simulink model "mrefrobotarm_modified_previous_y_previous_u_previous_ref_pert"  (R2018b)
settings: Solver=FixedStepAuto  StartTime=0.0  StopTime=10  RelTol=1e-3  AbsTol=1e-6
undefined symbols (not defined in the file or in its folder): cc, options
libraries: neural x714, simulink x1
(part 6 of 26)

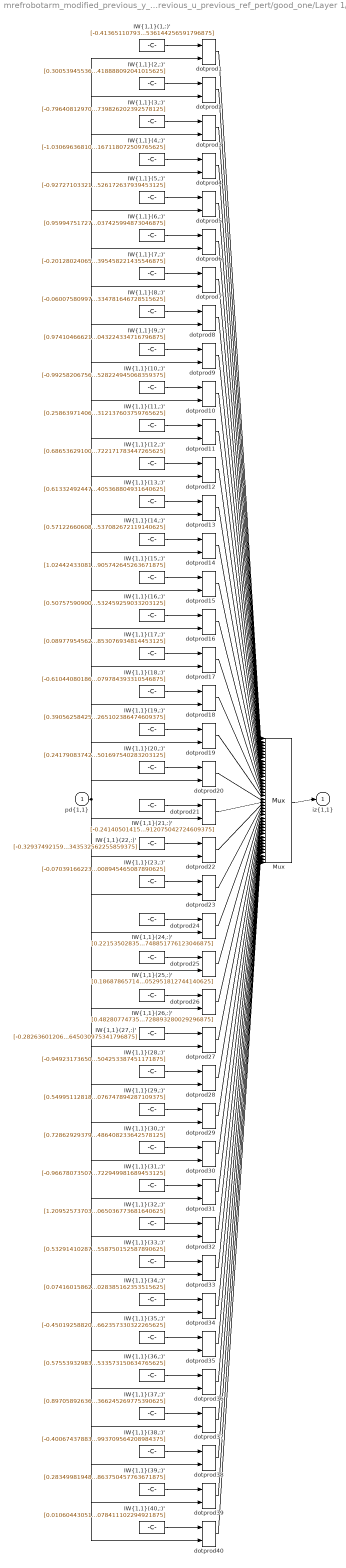
== system mrefrobotarm_modified_previous_y_previous_u_previous_ref_pert/good_one/Layer 1/IW{1,1} ==
  "pd{1,1}" : Inport  PortDimensions=10
      mask Display: e = 0.06;c1 = [120 230 180]/255;c2 = ([120 230 180]+0)/(256+128);c3 = ([120 230 180]+128)/(256+128);patch([0 1 1 0],[0 0 1 1],c1);patch([0 1 1 1-e 1-e 0+e],[0 0 1 1-e 0+e 0+e],c2);patch([0 0 1 1-e 0+e 0+e],[0 1 1 1-e 1-e 0+e],c3);plot([0 1 1 0 0],[0 0 1 1 0]);
  "IW{1,1}(1,:)'" : Constant  Value=[-0.413651107935018635952673093925113789737224578857421875;0.3836269510828476114738805335946381092071533203125;0.50232710069936759023079275721102021634578704833984375;-1.000665970829996087587687725317664444446563720703125;-0.1542635339068328670375507272183313034474849700927734375;-0.8218009806009398676707178310607559978961944580078125;-0.417486068359214090861541990307159721851348876953125;0.867526729012368047477821164648048579692840576171875;-0.98301388214653051544900108638103120028972625732421875;-0.0193724473873694395809064161539936321787536144256591796875]
      mask Display: e = 0.06;c1 = [120 150 230]/255;c2 = ([120 150 230]+0)/383;c3 = ([120 150 230]+128)/383;patch([0 1 1 0],[0 0 1 1],c1);patch([0 1 1 1-e 1-e 0+e],[0 0 1 1-e 0+e 0+e],c2);patch([0 0 1 1-e 0+e 0+e],[0 1 1 1-e 1-e 0+e],c3);plot([0 1 1 0 0],[0 0 1 1 0]);disp('Weights');
  "IW{1,1}(10,:)'" : Constant  Value=[-0.9925820675659589031880614129477180540561676025390625;0.2409702921885312765226672127027995884418487548828125;0.052011920879238393577992383143282495439052581787109375;-0.416376750462584432899149078366463072597980499267578125;-0.96039113919741703195853688157512806355953216552734375;0.62063415478920413992369731204234994947910308837890625;-0.8630530306659343064978884285665117204189300537109375;0.60936291205421666550279269358725287020206451416015625;-0.09827055594646873226682970425827079452574253082275390625;0.488985628143102812881437557734898291528224945068359375]
      mask Display: e = 0.06;c1 = [120 150 230]/255;c2 = ([120 150 230]+0)/383;c3 = ([120 150 230]+128)/383;patch([0 1 1 0],[0 0 1 1],c1);patch([0 1 1 1-e 1-e 0+e],[0 0 1 1-e 0+e 0+e],c2);patch([0 0 1 1-e 0+e 0+e],[0 1 1 1-e 1-e 0+e],c3);plot([0 1 1 0 0],[0 0 1 1 0]);disp('Weights');
  "IW{1,1}(11,:)'" : Constant  Value=[0.2586397140629539403988701451453380286693572998046875;-0.82856549831495229785360834284801967442035675048828125;0.6264712959270088976637680389103479683399200439453125;0.75547506719408696884698883877717889845371246337890625;0.59640906838833218639450706177740357816219329833984375;-0.785029365476563878445404043304733932018280029296875;-0.347310950192660339297390237334184348583221435546875;-0.462157651619720721836159782469621859490871429443359375;-1.1325499249033577076062329069827683269977569580078125;0.3696119827837540672277327757910825312137603759765625]
      mask Display: e = 0.06;c1 = [120 150 230]/255;c2 = ([120 150 230]+0)/383;c3 = ([120 150 230]+128)/383;patch([0 1 1 0],[0 0 1 1],c1);patch([0 1 1 1-e 1-e 0+e],[0 0 1 1-e 0+e 0+e],c2);patch([0 0 1 1-e 0+e 0+e],[0 1 1 1-e 1-e 0+e],c3);plot([0 1 1 0 0],[0 0 1 1 0]);disp('Weights');
  "IW{1,1}(12,:)'" : Constant  Value=[0.68653629100552582276151269979891367256641387939453125;-0.0248886322461292323893200517659352044574916362762451171875;0.447180501328404200744870422568055801093578338623046875;-0.44198123420568524721829817281104624271392822265625;-1.2490651394449863165192482483689673244953155517578125;0.4830653108523133010265837583574466407299041748046875;-0.392759951245398808428177517271251417696475982666015625;0.1335766512357776936159581282481667585670948028564453125;-0.583482604222464118493007845245301723480224609375;0.500678183603759041631064974353648722171783447265625]
      mask Display: e = 0.06;c1 = [120 150 230]/255;c2 = ([120 150 230]+0)/383;c3 = ([120 150 230]+128)/383;patch([0 1 1 0],[0 0 1 1],c1);patch([0 1 1 1-e 1-e 0+e],[0 0 1 1-e 0+e 0+e],c2);patch([0 0 1 1-e 0+e 0+e],[0 1 1 1-e 1-e 0+e],c3);plot([0 1 1 0 0],[0 0 1 1 0]);disp('Weights');
  "IW{1,1}(13,:)'" : Constant  Value=[0.6133249244779575004571370300254784524440765380859375;0.2368863057068739952359948119919863529503345489501953125;-0.826730624883238451872102814377285540103912353515625;-0.81502965756012690778931073509738780558109283447265625;0.049822669627226069677394804102732450701296329498291015625;0.49182006191557137153580470112501643598079681396484375;0.067178707635307921552936250009224750101566314697265625;0.145702225927659856363760582098620943725109100341796875;0.230253060188553015930068568195565603673458099365234375;1.0194493979983862974592057071276940405368804931640625]
      mask Display: e = 0.06;c1 = [120 150 230]/255;c2 = ([120 150 230]+0)/383;c3 = ([120 150 230]+128)/383;patch([0 1 1 0],[0 0 1 1],c1);patch([0 1 1 1-e 1-e 0+e],[0 0 1 1-e 0+e 0+e],c2);patch([0 0 1 1-e 0+e 0+e],[0 1 1 1-e 1-e 0+e],c3);plot([0 1 1 0 0],[0 0 1 1 0]);disp('Weights');
  "IW{1,1}(14,:)'" : Constant  Value=[0.57122660608382125335680257194326259195804595947265625;-0.70113249391813214916879815064021386206150054931640625;-0.0086478499608871224613171335704464581795036792755126953125;0.5990449634267556167088741858606226742267608642578125;-0.0532433606170133189028348397187073715031147003173828125;0.95479246182017474264824841156951151788234710693359375;-0.67799642096428913706773755620815791189670562744140625;0.157662545375461260466209978403639979660511016845703125;0.47531924881363696311353805867838673293590545654296875;1.1223503909760312868826304111280478537082672119140625]
      mask Display: e = 0.06;c1 = [120 150 230]/255;c2 = ([120 150 230]+0)/383;c3 = ([120 150 230]+128)/383;patch([0 1 1 0],[0 0 1 1],c1);patch([0 1 1 1-e 1-e 0+e],[0 0 1 1-e 0+e 0+e],c2);patch([0 0 1 1-e 0+e 0+e],[0 1 1 1-e 1-e 0+e],c3);plot([0 1 1 0 0],[0 0 1 1 0]);disp('Weights');
  "IW{1,1}(15,:)'" : Constant  Value=[1.024424330811316341538486085482873022556304931640625;-0.11900181038713032732889729459202499128878116607666015625;-0.89301318009671770692392556156846694648265838623046875;0.286811956595100336908643612332525663077831268310546875;0.9562237123416152950738933213870041072368621826171875;0.66112349620669796923522198994760401546955108642578125;0.65942560869206012785781467755441553890705108642578125;-0.3635154948717345124720168314524926245212554931640625;-0.12615629404641903743566899720462970435619354248046875;0.1510476304024055138608417792056570760905742645263671875]
      mask Display: e = 0.06;c1 = [120 150 230]/255;c2 = ([120 150 230]+0)/383;c3 = ([120 150 230]+128)/383;patch([0 1 1 0],[0 0 1 1],c1);patch([0 1 1 1-e 1-e 0+e],[0 0 1 1-e 0+e 0+e],c2);patch([0 0 1 1-e 0+e 0+e],[0 1 1 1-e 1-e 0+e],c3);plot([0 1 1 0 0],[0 0 1 1 0]);disp('Weights');
  "IW{1,1}(16,:)'" : Constant  Value=[0.50757590900584437232367918113595806062221527099609375;-0.68550796743866182492155303407344035804271697998046875;0.845989680309202629615583646227605640888214111328125;-0.301001414510317422124074937528348527848720550537109375;-0.5131342658860080785387935975450091063976287841796875;0.55499089075900476242253489544964395463466644287109375;0.87265805917673666680656197058851830661296844482421875;0.56120439816466494153957000889931805431842803955078125;0.3991413846511429053265374022885225713253021240234375;0.58399825658444382003864348007482476532459259033203125]
      mask Display: e = 0.06;c1 = [120 150 230]/255;c2 = ([120 150 230]+0)/383;c3 = ([120 150 230]+128)/383;patch([0 1 1 0],[0 0 1 1],c1);patch([0 1 1 1-e 1-e 0+e],[0 0 1 1-e 0+e 0+e],c2);patch([0 0 1 1-e 0+e 0+e],[0 1 1 1-e 1-e 0+e],c3);plot([0 1 1 0 0],[0 0 1 1 0]);disp('Weights');
  "IW{1,1}(17,:)'" : Constant  Value=[0.08977954562821359452140512757978285662829875946044921875;0.450162042402085627035290826825075782835483551025390625;-0.277132842312844906995650262615527026355266571044921875;-0.89533484630924953240338481919025070965290069580078125;0.48814571614230484186691683134995400905609130859375;-0.62095272399335910140649730237782932817935943603515625;-0.45038353462766200774325398015207611024379730224609375;-0.49284862337333013027063088884460739791393280029296875;0.760357222341462968273617661907337605953216552734375;0.70640094347899140547752949714777059853076934814453125]
      mask Display: e = 0.06;c1 = [120 150 230]/255;c2 = ([120 150 230]+0)/383;c3 = ([120 150 230]+128)/383;patch([0 1 1 0],[0 0 1 1],c1);patch([0 1 1 1-e 1-e 0+e],[0 0 1 1-e 0+e 0+e],c2);patch([0 0 1 1-e 0+e 0+e],[0 1 1 1-e 1-e 0+e],c3);plot([0 1 1 0 0],[0 0 1 1 0]);disp('Weights');
  "IW{1,1}(18,:)'" : Constant  Value=[-0.6104408018694840176721072566579096019268035888671875;-1.0336913526824804687720416040974669158458709716796875;0.270725265822102378887592522005434148013591766357421875;-0.380750786613607061781294760294258594512939453125;0.33268512528966043273470631902455352246761322021484375;-1.001093745459246786566609443980269134044647216796875;0.158315525907221921197987057894351892173290252685546875;-0.53153054346245409700344453085563145577907562255859375;-0.7668902743210084249625424490659497678279876708984375;-0.16671042993793416808756546743097715079784393310546875]
      mask Display: e = 0.06;c1 = [120 150 230]/255;c2 = ([120 150 230]+0)/383;c3 = ([120 150 230]+128)/383;patch([0 1 1 0],[0 0 1 1],c1);patch([0 1 1 1-e 1-e 0+e],[0 0 1 1-e 0+e 0+e],c2);patch([0 0 1 1-e 0+e 0+e],[0 1 1 1-e 1-e 0+e],c3);plot([0 1 1 0 0],[0 0 1 1 0]);disp('Weights');
  "IW{1,1}(19,:)'" : Constant  Value=[0.3905625842580298101580638103769160807132720947265625;0.0308098706564870587765181397799096885137259960174560546875;0.062138100461527102924552679041880764998495578765869140625;0.622615013248140058976787258870899677276611328125;0.99643920501872529360554153754492290318012237548828125;0.618145409712675064639597621862776577472686767578125;-1.1790025687618210792351192139904014766216278076171875;0.43713177654620272161167804370052181184291839599609375;-0.1320814385678981406346821358965826220810413360595703125;0.63245679741952220975775844635791145265102386474609375]
      mask Display: e = 0.06;c1 = [120 150 230]/255;c2 = ([120 150 230]+0)/383;c3 = ([120 150 230]+128)/383;patch([0 1 1 0],[0 0 1 1],c1);patch([0 1 1 1-e 1-e 0+e],[0 0 1 1-e 0+e 0+e],c2);patch([0 0 1 1-e 0+e 0+e],[0 1 1 1-e 1-e 0+e],c3);plot([0 1 1 0 0],[0 0 1 1 0]);disp('Weights');
  "IW{1,1}(2,:)'" : Constant  Value=[0.30053945536555570772208056951058097183704376220703125;0.481520714463711529962353097289451397955417633056640625;0.32855722206039239541297547475551255047321319580078125;-1.023620353434349983245965631795115768909454345703125;0.36139385403812862573857955794665031135082244873046875;-0.35510074464173346786566298760590143501758575439453125;0.53901574191551049342052692736615426838397979736328125;1.1478171331129953802729914968949742615222930908203125;0.01330999643922634555204265183192546828649938106536865234375;-0.8531970477840273847647267757565714418888092041015625]
      mask Display: e = 0.06;c1 = [120 150 230]/255;c2 = ([120 150 230]+0)/383;c3 = ([120 150 230]+128)/383;patch([0 1 1 0],[0 0 1 1],c1);patch([0 1 1 1-e 1-e 0+e],[0 0 1 1-e 0+e 0+e],c2);patch([0 0 1 1-e 0+e 0+e],[0 1 1 1-e 1-e 0+e],c3);plot([0 1 1 0 0],[0 0 1 1 0]);disp('Weights');
  "IW{1,1}(20,:)'" : Constant  Value=[0.2417908374206110544424319641620968468487262725830078125;-0.00914807597982341021147778548083806526847183704376220703125;0.084217128377931993465921323149814270436763763427734375;0.42983285451377406527484481557621620595455169677734375;1.3394232861488226671298207293148152530193328857421875;-0.381148886874808578983930829053861089050769805908203125;-0.1762973437296376510996509523465647362172603607177734375;0.09308197699677267511475520223029889166355133056640625;0.92227381408703601461951393503113649785518646240234375;1.077442550129131593195097593707032501697540283203125]
      mask Display: e = 0.06;c1 = [120 150 230]/255;c2 = ([120 150 230]+0)/383;c3 = ([120 150 230]+128)/383;patch([0 1 1 0],[0 0 1 1],c1);patch([0 1 1 1-e 1-e 0+e],[0 0 1 1-e 0+e 0+e],c2);patch([0 0 1 1-e 0+e 0+e],[0 1 1 1-e 1-e 0+e],c3);plot([0 1 1 0 0],[0 0 1 1 0]);disp('Weights');
  "IW{1,1}(21,:)'" : Constant  Value=[-0.2414050141565159679490903954501845873892307281494140625;0.82367477414810907898612413191585801541805267333984375;-0.0105825294795365530686748201105729094706475734710693359375;0.1956113083766050919631851456870208494365215301513671875;-1.7069096984195322175281717136385850608348846435546875;1.0057780668058187156788108040927909314632415771484375;1.4591709688934726418807485970319248735904693603515625;-0.2593923279024730188524472396238707005977630615234375;0.41043551676310585651918927396764047443866729736328125;0.83741947098360502987901554661220870912075042724609375]
      mask Display: e = 0.06;c1 = [120 150 230]/255;c2 = ([120 150 230]+0)/383;c3 = ([120 150 230]+128)/383;patch([0 1 1 0],[0 0 1 1],c1);patch([0 1 1 1-e 1-e 0+e],[0 0 1 1-e 0+e 0+e],c2);patch([0 0 1 1-e 0+e 0+e],[0 1 1 1-e 1-e 0+e],c3);plot([0 1 1 0 0],[0 0 1 1 0]);disp('Weights');
  "IW{1,1}(22,:)'" : Constant  Value=[-0.32937492159880077391420627463958226144313812255859375;0.646622243844576782834110417752526700496673583984375;-0.02931361877227912915433449825286515988409519195556640625;0.436759612951945042080836856257519684731960296630859375;0.866285245725330721455748061998747289180755615234375;0.1793659302452613457656838136244914494454860687255859375;0.09031635641268757896948926600089180283248424530029296875;-0.5973200815445045552820602097199298441410064697265625;0.10267351667025111094933009781016153283417224884033203125;1.2656338190569369483995387781760655343532562255859375]
      mask Display: e = 0.06;c1 = [120 150 230]/255;c2 = ([120 150 230]+0)/383;c3 = ([120 150 230]+128)/383;patch([0 1 1 0],[0 0 1 1],c1);patch([0 1 1 1-e 1-e 0+e],[0 0 1 1-e 0+e 0+e],c2);patch([0 0 1 1-e 0+e 0+e],[0 1 1 1-e 1-e 0+e],c3);plot([0 1 1 0 0],[0 0 1 1 0]);disp('Weights');
  "IW{1,1}(23,:)'" : Constant  Value=[-0.0703916622397355862261747461161576211452484130859375;0.67191045082923650522133129925350658595561981201171875;-0.0242859635021656396214329021177036338485777378082275390625;-0.386628048517191180710739217829541303217411041259765625;-2.5074712136418124686088049202226102352142333984375;0.55235033890016993485261309615452773869037628173828125;0.74299364405580725634337113660876639187335968017578125;0.64206786309071850471497100443230010569095611572265625;-0.58043464748950912568403737168409861624240875244140625;-0.422889498711053912760604589493595995008945465087890625]
      mask Display: e = 0.06;c1 = [120 150 230]/255;c2 = ([120 150 230]+0)/383;c3 = ([120 150 230]+128)/383;patch([0 1 1 0],[0 0 1 1],c1);patch([0 1 1 1-e 1-e 0+e],[0 0 1 1-e 0+e 0+e],c2);patch([0 0 1 1-e 0+e 0+e],[0 1 1 1-e 1-e 0+e],c3);plot([0 1 1 0 0],[0 0 1 1 0]);disp('Weights');
  "IW{1,1}(24,:)'" : Constant  Value=[0.221535028351505680621613691982929594814777374267578125;-0.8698822208881937800839523333706893026828765869140625;-0.2182601953161487917665084523832774721086025238037109375;0.4079298497457213290573463382315821945667266845703125;-0.36144550181965640067716094563365913927555084228515625;-0.28639131544193630052319576861918903887271881103515625;0.9540574961812564591667751301429234445095062255859375;-0.28396445607271247890679433112381957471370697021484375;0.364127425092508449910866374921170063316822052001953125;-0.004278262852394447250670150850737627479247748851776123046875]
      mask Display: e = 0.06;c1 = [120 150 230]/255;c2 = ([120 150 230]+0)/383;c3 = ([120 150 230]+128)/383;patch([0 1 1 0],[0 0 1 1],c1);patch([0 1 1 1-e 1-e 0+e],[0 0 1 1-e 0+e 0+e],c2);patch([0 0 1 1-e 0+e 0+e],[0 1 1 1-e 1-e 0+e],c3);plot([0 1 1 0 0],[0 0 1 1 0]);disp('Weights');
  "IW{1,1}(25,:)'" : Constant  Value=[0.186878657149024240968770982362912036478519439697265625;-0.7759331943091141159385415448923595249652862548828125;0.2148465953621268298423530040963669307529926300048828125;-0.92201175425662285078942659310996532440185546875;0.59498484563237952205128067362238653004169464111328125;-0.66139341790903605211582316769636236131191253662109375;0.67596601108655107736922218464314937591552734375;-0.458533778996277507911116799732553772628307342529296875;-0.322071301367099327439547096219030208885669708251953125;0.8937721561967253425251556109287776052951812744140625]
      mask Display: e = 0.06;c1 = [120 150 230]/255;c2 = ([120 150 230]+0)/383;c3 = ([120 150 230]+128)/383;patch([0 1 1 0],[0 0 1 1],c1);patch([0 1 1 1-e 1-e 0+e],[0 0 1 1-e 0+e 0+e],c2);patch([0 0 1 1-e 0+e 0+e],[0 1 1 1-e 1-e 0+e],c3);plot([0 1 1 0 0],[0 0 1 1 0]);disp('Weights');
  "IW{1,1}(26,:)'" : Constant  Value=[0.482807747351104932231891098126652650535106658935546875;-0.274643538698023714772489256574772298336029052734375;0.977117390542808994524648369406349956989288330078125;-0.72784044851192764014058411703445017337799072265625;-0.298911347579471187163591139324125833809375762939453125;-0.351550652031840493716430273707373999059200286865234375;-0.7121513278393643009422930845175869762897491455078125;0.94265145728446686490542560932226479053497314453125;-0.63767361421792767561811388077330775558948516845703125;-0.465068595673045592775451950728893280029296875]
      mask Display: e = 0.06;c1 = [120 150 230]/255;c2 = ([120 150 230]+0)/383;c3 = ([120 150 230]+128)/383;patch([0 1 1 0],[0 0 1 1],c1);patch([0 1 1 1-e 1-e 0+e],[0 0 1 1-e 0+e 0+e],c2);patch([0 0 1 1-e 0+e 0+e],[0 1 1 1-e 1-e 0+e],c3);plot([0 1 1 0 0],[0 0 1 1 0]);disp('Weights');
  "IW{1,1}(27,:)'" : Constant  Value=[-0.2826360120640381001777541314368136227130889892578125;1.0331384188045353855756047778413631021976470947265625;0.2538275640105565056359182563028298318386077880859375;-0.6876811465011194446361741938744671642780303955078125;0.4368710842237082392358615834382362663745880126953125;0.476320854183213071575409003344248048961162567138671875;0.443648508004234332080528702135779894888401031494140625;-0.62347776206357463646412497837445698678493499755859375;0.43560219075936379429236922078416682779788970947265625;0.6740756065088635562432273218291811645030975341796875]
      mask Display: e = 0.06;c1 = [120 150 230]/255;c2 = ([120 150 230]+0)/383;c3 = ([120 150 230]+128)/383;patch([0 1 1 0],[0 0 1 1],c1);patch([0 1 1 1-e 1-e 0+e],[0 0 1 1-e 0+e 0+e],c2);patch([0 0 1 1-e 0+e 0+e],[0 1 1 1-e 1-e 0+e],c3);plot([0 1 1 0 0],[0 0 1 1 0]);disp('Weights');
  "IW{1,1}(28,:)'" : Constant  Value=[-0.94923173650253056532477557993843220174312591552734375;-0.98442046864123933236356833731406368315219879150390625;0.41376330233902114397182003813213668763637542724609375;0.439113670992825666505865456201718188822269439697265625;0.21542815920926638995069879456423223018646240234375;-0.93574938767304816078507201382308267056941986083984375;0.787753205288106439496687016799114644527435302734375;-0.226104675231449281369577875011600553989410400390625;0.048265716907905320542937488426105119287967681884765625;0.54952586236559042287552756533841602504253387451171875]
      mask Display: e = 0.06;c1 = [120 150 230]/255;c2 = ([120 150 230]+0)/383;c3 = ([120 150 230]+128)/383;patch([0 1 1 0],[0 0 1 1],c1);patch([0 1 1 1-e 1-e 0+e],[0 0 1 1-e 0+e 0+e],c2);patch([0 0 1 1-e 0+e 0+e],[0 1 1 1-e 1-e 0+e],c3);plot([0 1 1 0 0],[0 0 1 1 0]);disp('Weights');
  "IW{1,1}(29,:)'" : Constant  Value=[0.54995112818424851663934305179282091557979583740234375;-0.96548476888214762592355100423446856439113616943359375;-0.6133643858887316557826352436677552759647369384765625;-0.369747278830332037902195452261366881430149078369140625;-0.4889943619153596099380365558317862451076507568359375;-0.4574687563627983788450137581094168126583099365234375;-0.9918414740130405693463444549706764519214630126953125;-0.439705044341271389374270484040607698261737823486328125;0.5677934762199841056684590512304566800594329833984375;-0.5441783375664319688524983575916849076747894287109375]
      mask Display: e = 0.06;c1 = [120 150 230]/255;c2 = ([120 150 230]+0)/383;c3 = ([120 150 230]+128)/383;patch([0 1 1 0],[0 0 1 1],c1);patch([0 1 1 1-e 1-e 0+e],[0 0 1 1-e 0+e 0+e],c2);patch([0 0 1 1-e 0+e 0+e],[0 1 1 1-e 1-e 0+e],c3);plot([0 1 1 0 0],[0 0 1 1 0]);disp('Weights');
  "IW{1,1}(3,:)'" : Constant  Value=[-0.79640812970941443627026501417276449501514434814453125;-0.96725622206039030270829925939324311912059783935546875;-0.81005379713580738521017110542743466794490814208984375;0.07789219319437627742086505122642847709357738494873046875;-0.86489171738730241667525433513219468295574188232421875;0.81312859030495265866278487010276876389980316162109375;-0.12379626000382269734867435317937633953988552093505859375;-0.6992501943224880278648925013840198516845703125;-0.0202103147915163768033597335715967346914112567901611328125;0.4651949651069664515290469353203661739826202392578125]
      mask Display: e = 0.06;c1 = [120 150 230]/255;c2 = ([120 150 230]+0)/383;c3 = ([120 150 230]+128)/383;patch([0 1 1 0],[0 0 1 1],c1);patch([0 1 1 1-e 1-e 0+e],[0 0 1 1-e 0+e 0+e],c2);patch([0 0 1 1-e 0+e 0+e],[0 1 1 1-e 1-e 0+e],c3);plot([0 1 1 0 0],[0 0 1 1 0]);disp('Weights');
  "IW{1,1}(30,:)'" : Constant  Value=[0.72862929379874075141998446270008571445941925048828125;0.57099515174563386654682517473702318966388702392578125;-0.09992527021377718698946779340985813178122043609619140625;0.411812398181885364056853404690627939999103546142578125;-1.1646039332940241184388696638052351772785186767578125;-0.81635251644773576540359272257774136960506439208984375;-0.1168473553190165492576824135539936833083629608154296875;-0.359766465525852507933990409583202563226222991943359375;0.6195063284556125982049934464157558977603912353515625;0.038312220849707818992602170737882261164486408233642578125]
      mask Display: e = 0.06;c1 = [120 150 230]/255;c2 = ([120 150 230]+0)/383;c3 = ([120 150 230]+128)/383;patch([0 1 1 0],[0 0 1 1],c1);patch([0 1 1 1-e 1-e 0+e],[0 0 1 1-e 0+e 0+e],c2);patch([0 0 1 1-e 0+e 0+e],[0 1 1 1-e 1-e 0+e],c3);plot([0 1 1 0 0],[0 0 1 1 0]);disp('Weights');
  "IW{1,1}(31,:)'" : Constant  Value=[-0.96678073507359851834763730948907323181629180908203125;0.09148655759019690136835123439595918171107769012451171875;0.709549141602580757393070598482154309749603271484375;-0.410248808800185826850537296195398084819316864013671875;-0.7370652145869300841951599068124778568744659423828125;-0.438942207461164246584672810058691538870334625244140625;-0.80989777442946098151566047818050719797611236572265625;0.94874940597907764239238304071477614343166351318359375;0.2334139145840961881983588455113931559026241302490234375;0.405630960838893106501501506500062532722949981689453125]
      mask Display: e = 0.06;c1 = [120 150 230]/255;c2 = ([120 150 230]+0)/383;c3 = ([120 150 230]+128)/383;patch([0 1 1 0],[0 0 1 1],c1);patch([0 1 1 1-e 1-e 0+e],[0 0 1 1-e 0+e 0+e],c2);patch([0 0 1 1-e 0+e 0+e],[0 1 1 1-e 1-e 0+e],c3);plot([0 1 1 0 0],[0 0 1 1 0]);disp('Weights');
  "IW{1,1}(32,:)'" : Constant  Value=[1.2095257370328458268460281033185310661792755126953125;0.35065561767196407050306561359320767223834991455078125;-0.95698055747720101038567008799873292446136474609375;-0.18743931116112688695096721858135424554347991943359375;-1.0822736049319747753116871535894460976123809814453125;1.075874990384995566472525752033106982707977294921875;-0.352754600872055512628122642126982100307941436767578125;0.314480530229425181421021306960028596222400665283203125;-1.20745251513363083262220243341289460659027099609375;0.134532970678878316395099545843550004065036773681640625]
      mask Display: e = 0.06;c1 = [120 150 230]/255;c2 = ([120 150 230]+0)/383;c3 = ([120 150 230]+128)/383;patch([0 1 1 0],[0 0 1 1],c1);patch([0 1 1 1-e 1-e 0+e],[0 0 1 1-e 0+e 0+e],c2);patch([0 0 1 1-e 0+e 0+e],[0 1 1 1-e 1-e 0+e],c3);plot([0 1 1 0 0],[0 0 1 1 0]);disp('Weights');
  "IW{1,1}(33,:)'" : Constant  Value=[0.532914102879858742056740084080956876277923583984375;1.105100254369091317130369134247303009033203125;0.87151392502779201354456972694606520235538482666015625;0.2321724557656669463145959753092029131948947906494140625;0.1575035363103396424122593089123256504535675048828125;0.303249717909266192084061231071245856583118438720703125;0.2212907592801952871841564274291158653795719146728515625;0.31905523329310703228856027635629288852214813232421875;0.9408906635522378270053422966157086193561553955078125;0.293277365914686394265942226411425508558750152587890625]
      mask Display: e = 0.06;c1 = [120 150 230]/255;c2 = ([120 150 230]+0)/383;c3 = ([120 150 230]+128)/383;patch([0 1 1 0],[0 0 1 1],c1);patch([0 1 1 1-e 1-e 0+e],[0 0 1 1-e 0+e 0+e],c2);patch([0 0 1 1-e 0+e 0+e],[0 1 1 1-e 1-e 0+e],c3);plot([0 1 1 0 0],[0 0 1 1 0]);disp('Weights');
  "IW{1,1}(34,:)'" : Constant  Value=[0.07416015862654136425735629245536983944475650787353515625;-1.0397513415756154397939781119930557906627655029296875;-0.04961495021440388841771351735587813891470432281494140625;-0.38815439020895003974231940446770749986171722412109375;-0.731899181421933775482102646492421627044677734375;0.47747292946845687477974706780514679849147796630859375;0.54281059692801625349289906807825900614261627197265625;-0.3797969606031086353681303080520592629909515380859375;0.6361926650398481708492681718780659139156341552734375;-0.81464825546781993725886650281609036028385162353515625]
      mask Display: e = 0.06;c1 = [120 150 230]/255;c2 = ([120 150 230]+0)/383;c3 = ([120 150 230]+128)/383;patch([0 1 1 0],[0 0 1 1],c1);patch([0 1 1 1-e 1-e 0+e],[0 0 1 1-e 0+e 0+e],c2);patch([0 0 1 1-e 0+e 0+e],[0 1 1 1-e 1-e 0+e],c3);plot([0 1 1 0 0],[0 0 1 1 0]);disp('Weights');
  "IW{1,1}(35,:)'" : Constant  Value=[-0.450192588202033838751248140397365204989910125732421875;-0.99347786502311230538708741732989437878131866455078125;-0.1129298144360480760095555297084501944482326507568359375;0.81995183619318823264876527900923974812030792236328125;-0.0285397314603526054688220625621397630311548709869384765625;-0.65224530055292107011410962513764388859272003173828125;-0.96858801591490106819293259832193143665790557861328125;-0.71417961178618316608890381758101284503936767578125;-0.050839792046079086695886672941924189217388629913330078125;-0.58702131782338773380303109661326743662357330322265625]
      mask Display: e = 0.06;c1 = [120 150 230]/255;c2 = ([120 150 230]+0)/383;c3 = ([120 150 230]+128)/383;patch([0 1 1 0],[0 0 1 1],c1);patch([0 1 1 1-e 1-e 0+e],[0 0 1 1-e 0+e 0+e],c2);patch([0 0 1 1-e 0+e 0+e],[0 1 1 1-e 1-e 0+e],c3);plot([0 1 1 0 0],[0 0 1 1 0]);disp('Weights');
  "IW{1,1}(36,:)'" : Constant  Value=[0.57553932983433464531941581299179233610630035400390625;0.56717154016443915853784574210294522345066070556640625;0.62350177817309770933462687025894410908222198486328125;0.67306586104355015098832382136606611311435699462890625;0.5984586458511629292189581974525935947895050048828125;-0.984305982041815408223328631720505654811859130859375;0.396982307671666700965573681969544850289821624755859375;0.7717145366065356615337123002973385155200958251953125;-0.337280702863450410067258644630783237516880035400390625;0.050723155982260570429076551590696908533573150634765625]
      mask Display: e = 0.06;c1 = [120 150 230]/255;c2 = ([120 150 230]+0)/383;c3 = ([120 150 230]+128)/383;patch([0 1 1 0],[0 0 1 1],c1);patch([0 1 1 1-e 1-e 0+e],[0 0 1 1-e 0+e 0+e],c2);patch([0 0 1 1-e 0+e 0+e],[0 1 1 1-e 1-e 0+e],c3);plot([0 1 1 0 0],[0 0 1 1 0]);disp('Weights');
  "IW{1,1}(37,:)'" : Constant  Value=[0.8970589263675419200438909683725796639919281005859375;-0.613332686523948122925276038586162030696868896484375;-1.2203901910177084033648498007096350193023681640625;0.3569428745995850693617512661148793995380401611328125;-0.10171219534107354964813652031807578168809413909912109375;0.272452491953151521020259906435967423021793365478515625;-0.5628059414309660724029527045786380767822265625;-1.0797282369090737130790103037725202739238739013671875;-0.66145317648137413879538826222415082156658172607421875;-0.207414645751535398066067727995687164366245269775390625]
      mask Display: e = 0.06;c1 = [120 150 230]/255;c2 = ([120 150 230]+0)/383;c3 = ([120 150 230]+128)/383;patch([0 1 1 0],[0 0 1 1],c1);patch([0 1 1 1-e 1-e 0+e],[0 0 1 1-e 0+e 0+e],c2);patch([0 0 1 1-e 0+e 0+e],[0 1 1 1-e 1-e 0+e],c3);plot([0 1 1 0 0],[0 0 1 1 0]);disp('Weights');
  "IW{1,1}(38,:)'" : Constant  Value=[-0.40067437883748102667169632695731706917285919189453125;-0.57670391675015497678913334311801008880138397216796875;0.41049531478886713831144561481778509914875030517578125;0.822781172118504766643809489323757588863372802734375;-0.604369306380508231058001911151222884654998779296875;-0.77865645392512938816054202106897719204425811767578125;0.76106556238663947144829080571071244776248931884765625;0.61141666686727325075167982504353858530521392822265625;-0.25695930459092319875225030045839957892894744873046875;0.802452075891439076116284923045895993709564208984375]
      mask Display: e = 0.06;c1 = [120 150 230]/255;c2 = ([120 150 230]+0)/383;c3 = ([120 150 230]+128)/383;patch([0 1 1 0],[0 0 1 1],c1);patch([0 1 1 1-e 1-e 0+e],[0 0 1 1-e 0+e 0+e],c2);patch([0 0 1 1-e 0+e 0+e],[0 1 1 1-e 1-e 0+e],c3);plot([0 1 1 0 0],[0 0 1 1 0]);disp('Weights');
  "IW{1,1}(39,:)'" : Constant  Value=[0.283499819487878557122684242131072096526622772216796875;-0.94598333935438494446401591631001792848110198974609375;-0.1418727997506810112327002570964395999908447265625;0.9084104391468248440588695302722044289112091064453125;-0.36536748297059518097995578500558622181415557861328125;0.75533736854208755051587331763585098087787628173828125;0.67548606619028361830459061820874921977519989013671875;0.6661715911006613755063199278083629906177520751953125;0.1428603475355651186706751332167186774313449859619140625;0.50410242781748137996800096516381017863750457763671875]
      mask Display: e = 0.06;c1 = [120 150 230]/255;c2 = ([120 150 230]+0)/383;c3 = ([120 150 230]+128)/383;patch([0 1 1 0],[0 0 1 1],c1);patch([0 1 1 1-e 1-e 0+e],[0 0 1 1-e 0+e 0+e],c2);patch([0 0 1 1-e 0+e 0+e],[0 1 1 1-e 1-e 0+e],c3);plot([0 1 1 0 0],[0 0 1 1 0]);disp('Weights');
  "IW{1,1}(4,:)'" : Constant  Value=[-1.030696368109789151645827587344683706760406494140625;0.80375696330114509979836157071986235678195953369140625;-0.61921159358025856800367137111607007682323455810546875;0.315224798578327025655454463048954494297504425048828125;0.334295259389772780878047342412173748016357421875;0.48787292962016481912002063836553134024143218994140625;-0.76385573944577134231082027326920069754123687744140625;0.12038173141899420615086313546271412633359432220458984375;0.43555551494740896156798726224224083125591278076171875;0.5205510485425739464204752948717214167118072509765625]
      mask Display: e = 0.06;c1 = [120 150 230]/255;c2 = ([120 150 230]+0)/383;c3 = ([120 150 230]+128)/383;patch([0 1 1 0],[0 0 1 1],c1);patch([0 1 1 1-e 1-e 0+e],[0 0 1 1-e 0+e 0+e],c2);patch([0 0 1 1-e 0+e 0+e],[0 1 1 1-e 1-e 0+e],c3);plot([0 1 1 0 0],[0 0 1 1 0]);disp('Weights');
  "IW{1,1}(40,:)'" : Constant  Value=[0.01060443051167595136796695243219801341183483600616455078125;-0.0985956616986960465709444179083220660686492919921875;-0.397337087764881358165069968890747986733913421630859375;0.111049131410769941208371847096714191138744354248046875;-0.40798914215162429552918865738320164382457733154296875;0.01531768680549806978252735945034146425314247608184814453125;-1.1668017568985595833197521642432548105716705322265625;1.26328700686288453169936474296264350414276123046875;0.72747109799704856580859768655500374734401702880859375;-0.515334279793882910070124125923030078411102294921875]
      mask Display: e = 0.06;c1 = [120 150 230]/255;c2 = ([120 150 230]+0)/383;c3 = ([120 150 230]+128)/383;patch([0 1 1 0],[0 0 1 1],c1);patch([0 1 1 1-e 1-e 0+e],[0 0 1 1-e 0+e 0+e],c2);patch([0 0 1 1-e 0+e 0+e],[0 1 1 1-e 1-e 0+e],c3);plot([0 1 1 0 0],[0 0 1 1 0]);disp('Weights');
  "IW{1,1}(5,:)'" : Constant  Value=[-0.92727103321418835601974706150940619409084320068359375;0.44379942056044530129810254948097281157970428466796875;0.338606926976893485292663399377488531172275543212890625;0.7947964648923793173906915399129502475261688232421875;-0.169057435849373494107794613228179514408111572265625;-0.356381664950746246400825611999607644975185394287109375;0.305277014866351892319329408564954064786434173583984375;0.7891281326524353101348197014885954558849334716796875;0.18661985730503893865517284211819060146808624267578125;0.7481044654260433635073468394693918526172637939453125]
      mask Display: e = 0.06;c1 = [120 150 230]/255;c2 = ([120 150 230]+0)/383;c3 = ([120 150 230]+128)/383;patch([0 1 1 0],[0 0 1 1],c1);patch([0 1 1 1-e 1-e 0+e],[0 0 1 1-e 0+e 0+e],c2);patch([0 0 1 1-e 0+e 0+e],[0 1 1 1-e 1-e 0+e],c3);plot([0 1 1 0 0],[0 0 1 1 0]);disp('Weights');
  "IW{1,1}(6,:)'" : Constant  Value=[0.9599475172783498155837378362775780260562896728515625;0.37862864056876011087382494224584661424160003662109375;-0.4503091139884158877748632221482694149017333984375;0.64762803856415473990892905931104905903339385986328125;-0.488601817347305289462866539906826801598072052001953125;-0.79221204669759692773567394397105090320110321044921875;0.94355183029172173814203006259049288928508758544921875;0.533269505938972709913059588870964944362640380859375;-0.1182119914878387856305153036373667418956756591796875;0.57225674445003704704504343681037425994873046875]
      mask Display: e = 0.06;c1 = [120 150 230]/255;c2 = ([120 150 230]+0)/383;c3 = ([120 150 230]+128)/383;patch([0 1 1 0],[0 0 1 1],c1);patch([0 1 1 1-e 1-e 0+e],[0 0 1 1-e 0+e 0+e],c2);patch([0 0 1 1-e 0+e 0+e],[0 1 1 1-e 1-e 0+e],c3);plot([0 1 1 0 0],[0 0 1 1 0]);disp('Weights');
  "IW{1,1}(7,:)'" : Constant  Value=[-0.2012802406558749368503669074925710447132587432861328125;-0.168020637494278146650827920893789269030094146728515625;-0.5196267073941400749248487045406363904476165771484375;0.313752052912111889515500706693273968994617462158203125;-0.69539141795439018967073252497357316315174102783203125;-0.1551868567913933516511093557710410095751285552978515625;0.3783291165616986528874576833914034068584442138671875;-0.9846953608687252224029862190946005284786224365234375;0.54226114486496046485086708344169892370700836181640625;1.29434748139429967039859548094682395458221435546875]
      mask Display: e = 0.06;c1 = [120 150 230]/255;c2 = ([120 150 230]+0)/383;c3 = ([120 150 230]+128)/383;patch([0 1 1 0],[0 0 1 1],c1);patch([0 1 1 1-e 1-e 0+e],[0 0 1 1-e 0+e 0+e],c2);patch([0 0 1 1-e 0+e 0+e],[0 1 1 1-e 1-e 0+e],c3);plot([0 1 1 0 0],[0 0 1 1 0]);disp('Weights');
  "IW{1,1}(8,:)'" : Constant  Value=[-0.060075809978153038581893952141399495303630828857421875;0.97119678846992429921414213822572492063045501708984375;0.1757672395685068444937115827997331507503986358642578125;-0.24941681083479683156411965683219023048877716064453125;-0.09140453235137017962141925409014220349490642547607421875;-1.187514844774286704165433548041619360446929931640625;0.53757936663066541171929202391766011714935302734375;-0.333079409381347113505711377001716755330562591552734375;-0.61934089435207351215240123565308749675750732421875;0.502910850505925655085093239904381334781646728515625]
      mask Display: e = 0.06;c1 = [120 150 230]/255;c2 = ([120 150 230]+0)/383;c3 = ([120 150 230]+128)/383;patch([0 1 1 0],[0 0 1 1],c1);patch([0 1 1 1-e 1-e 0+e],[0 0 1 1-e 0+e 0+e],c2);patch([0 0 1 1-e 0+e 0+e],[0 1 1 1-e 1-e 0+e],c3);plot([0 1 1 0 0],[0 0 1 1 0]);disp('Weights');
  "IW{1,1}(9,:)'" : Constant  Value=[0.9741046662175241177550333304679952561855316162109375;-0.08659790627727402545499302277676179073750972747802734375;0.265979378087316142842411181845818646252155303955078125;-0.9553948679548092126623259900952689349651336669921875;-0.2071105243669991435861987838507047854363918304443359375;0.08764383733318670266498884302563965320587158203125;-0.595219368644193114192830762476660311222076416015625;0.64557065702977400878381786242243833839893341064453125;-0.57474207546024647097482329627382569015026092529296875;0.419022543348396669937727665455895476043224334716796875]
      mask Display: e = 0.06;c1 = [120 150 230]/255;c2 = ([120 150 230]+0)/383;c3 = ([120 150 230]+128)/383;patch([0 1 1 0],[0 0 1 1],c1);patch([0 1 1 1-e 1-e 0+e],[0 0 1 1-e 0+e 0+e],c2);patch([0 0 1 1-e 0+e 0+e],[0 1 1 1-e 1-e 0+e],c3);plot([0 1 1 0 0],[0 0 1 1 0]);disp('Weights');
  Mux : Mux  Inputs=40
      mask Display: e = 0.06;c1 = [120 150 230]/255;c2 = ([120 150 230]+0)/383;c3 = ([120 150 230]+128)/383;patch([0 1 1 0],[0 0 1 1],c1);patch([0 1 1 1-e 1-e 0+e],[0 0 1 1-e 0+e 0+e],c2);patch([0 0 1 1-e 0+e 0+e],[0 1 1 1-e 1-e 0+e],c3);plot([0 1 1 0 0],[0 0 1 1 0]);disp('Mux');
  dotprod{1..40} (40 alike) : neural/Weight Functions/dotprod
  "iz{1,1}" : Outport
      mask Display: e = 0.06;c1 = [120 230 180]/255;c2 = ([120 230 180]+0)/(256+128);c3 = ([120 230 180]+128)/(256+128);patch([0 1 1 0],[0 0 1 1],c1);patch([0 1 1 1-e 1-e 0+e],[0 0 1 1-e 0+e 0+e],c2);patch([0 0 1 1-e 0+e 0+e],[0 1 1 1-e 1-e 0+e],c3);plot([0 1 1 0 0],[0 0 1 1 0]);
  wires:
  "IW{1,1}(1,:)'"/1 -> dotprod1/1
  "pd{1,1}"/1 -> dotprod1/2, dotprod2/2, dotprod3/2, dotprod4/2, dotprod5/2, dotprod6/2, dotprod7/2, dotprod8/2, dotprod9/2, dotprod10/2, dotprod11/2, dotprod12/2, dotprod13/2, dotprod14/2, dotprod15/2, dotprod16/2, dotprod17/2, dotprod18/2, dotprod19/2, dotprod20/2, dotprod21/2, dotprod22/2, dotprod23/2, dotprod24/2, dotprod25/2, dotprod26/2, dotprod27/2, dotprod28/2, dotprod29/2, dotprod30/2, dotprod31/2, dotprod32/2, dotprod33/2, dotprod34/2, dotprod35/2, dotprod36/2, dotprod37/2, dotprod38/2, dotprod39/2, dotprod40/2
  dotprod1/1 -> Mux/1
  "IW{1,1}(2,:)'"/1 -> dotprod2/1
  dotprod2/1 -> Mux/2
  "IW{1,1}(3,:)'"/1 -> dotprod3/1
  dotprod3/1 -> Mux/3
  "IW{1,1}(4,:)'"/1 -> dotprod4/1
  dotprod4/1 -> Mux/4
  "IW{1,1}(5,:)'"/1 -> dotprod5/1
  dotprod5/1 -> Mux/5
  "IW{1,1}(6,:)'"/1 -> dotprod6/1
  dotprod6/1 -> Mux/6
  "IW{1,1}(7,:)'"/1 -> dotprod7/1
  dotprod7/1 -> Mux/7
  "IW{1,1}(8,:)'"/1 -> dotprod8/1
  dotprod8/1 -> Mux/8
  "IW{1,1}(9,:)'"/1 -> dotprod9/1
  dotprod9/1 -> Mux/9
  "IW{1,1}(10,:)'"/1 -> dotprod10/1
  dotprod10/1 -> Mux/10
  "IW{1,1}(11,:)'"/1 -> dotprod11/1
  dotprod11/1 -> Mux/11
  "IW{1,1}(12,:)'"/1 -> dotprod12/1
  dotprod12/1 -> Mux/12
  "IW{1,1}(13,:)'"/1 -> dotprod13/1
  dotprod13/1 -> Mux/13
  "IW{1,1}(14,:)'"/1 -> dotprod14/1
  dotprod14/1 -> Mux/14
  "IW{1,1}(15,:)'"/1 -> dotprod15/1
  dotprod15/1 -> Mux/15
  "IW{1,1}(16,:)'"/1 -> dotprod16/1
  dotprod16/1 -> Mux/16
  "IW{1,1}(17,:)'"/1 -> dotprod17/1
  dotprod17/1 -> Mux/17
  "IW{1,1}(18,:)'"/1 -> dotprod18/1
  dotprod18/1 -> Mux/18
  "IW{1,1}(19,:)'"/1 -> dotprod19/1
  dotprod19/1 -> Mux/19
  "IW{1,1}(20,:)'"/1 -> dotprod20/1
  dotprod20/1 -> Mux/20
  "IW{1,1}(21,:)'"/1 -> dotprod21/1
  dotprod21/1 -> Mux/21
  "IW{1,1}(22,:)'"/1 -> dotprod22/1
  dotprod22/1 -> Mux/22
  "IW{1,1}(23,:)'"/1 -> dotprod23/1
  dotprod23/1 -> Mux/23
  "IW{1,1}(24,:)'"/1 -> dotprod24/1
  dotprod24/1 -> Mux/24
  "IW{1,1}(25,:)'"/1 -> dotprod25/1
  dotprod25/1 -> Mux/25
  "IW{1,1}(26,:)'"/1 -> dotprod26/1
  dotprod26/1 -> Mux/26
  "IW{1,1}(27,:)'"/1 -> dotprod27/1
  dotprod27/1 -> Mux/27
  "IW{1,1}(28,:)'"/1 -> dotprod28/1
  dotprod28/1 -> Mux/28
  "IW{1,1}(29,:)'"/1 -> dotprod29/1
  dotprod29/1 -> Mux/29
  "IW{1,1}(30,:)'"/1 -> dotprod30/1
  dotprod30/1 -> Mux/30
  "IW{1,1}(31,:)'"/1 -> dotprod31/1
  dotprod31/1 -> Mux/31
  "IW{1,1}(32,:)'"/1 -> dotprod32/1
  dotprod32/1 -> Mux/32
  "IW{1,1}(33,:)'"/1 -> dotprod33/1
  dotprod33/1 -> Mux/33
  "IW{1,1}(34,:)'"/1 -> dotprod34/1
  dotprod34/1 -> Mux/34
  "IW{1,1}(35,:)'"/1 -> dotprod35/1
  dotprod35/1 -> Mux/35
  "IW{1,1}(36,:)'"/1 -> dotprod36/1
  dotprod36/1 -> Mux/36
  "IW{1,1}(37,:)'"/1 -> dotprod37/1
  dotprod37/1 -> Mux/37
  "IW{1,1}(38,:)'"/1 -> dotprod38/1
  dotprod38/1 -> Mux/38
  "IW{1,1}(39,:)'"/1 -> dotprod39/1
  dotprod39/1 -> Mux/39
  "IW{1,1}(40,:)'"/1 -> dotprod40/1
  dotprod40/1 -> Mux/40
  Mux/1 -> "iz{1,1}"/1

== system mrefrobotarm_modified_previous_y_previous_u_previous_ref_pert/good_one/Layer 2/Delays 1 ==
  "p{2}" : Inport  PortDimensions=40
      mask Display: e = 0.06;c1 = [120 230 180]/255;c2 = ([120 230 180]+0)/(256+128);c3 = ([120 230 180]+128)/(256+128);patch([0 1 1 0],[0 0 1 1],c1);patch([0 1 1 1-e 1-e 0+e],[0 0 1 1-e 0+e 0+e],c2);patch([0 0 1 1-e 0+e 0+e],[0 1 1 1-e 1-e 0+e],c3);plot([0 1 1 0 0],[0 0 1 1 0]);
  mux : Mux  Inputs=1
      mask Display: e = 0.06;c1 = [120 150 230]/255;c2 = ([120 150 230]+0)/383;c3 = ([120 150 230]+128)/383;patch([0 1 1 0],[0 0 1 1],c1);patch([0 1 1 1-e 1-e 0+e],[0 0 1 1-e 0+e 0+e],c2);patch([0 0 1 1-e 0+e 0+e],[0 1 1 1-e 1-e 0+e],c3);plot([0 1 1 0 0],[0 0 1 1 0]);disp('Mux')
  "pd{2,1}" : Outport
      mask Display: e = 0.06;c1 = [120 230 180]/255;c2 = ([120 230 180]+0)/(256+128);c3 = ([120 230 180]+128)/(256+128);patch([0 1 1 0],[0 0 1 1],c1);patch([0 1 1 1-e 1-e 0+e],[0 0 1 1-e 0+e 0+e],c2);patch([0 0 1 1-e 0+e 0+e],[0 1 1 1-e 1-e 0+e],c3);plot([0 1 1 0 0],[0 0 1 1 0]);
  wires:
  "p{2}"/1 -> mux/1
  mux/1 -> "pd{2,1}"/1

== system mrefrobotarm_modified_previous_y_previous_u_previous_ref_pert/good_one/Layer 2/LW{2,1} ==
  "ad{2,1}" : Inport  PortDimensions=40
      mask Display: e = 0.06;c1 = [120 230 180]/255;c2 = ([120 230 180]+0)/(256+128);c3 = ([120 230 180]+128)/(256+128);patch([0 1 1 0],[0 0 1 1],c1);patch([0 1 1 1-e 1-e 0+e],[0 0 1 1-e 0+e 0+e],c2);patch([0 0 1 1-e 0+e 0+e],[0 1 1 1-e 1-e 0+e],c3);plot([0 1 1 0 0],[0 0 1 1 0]);
  "IW{2,1}(1,:)'" : Constant  Value=[-0.016177229018260623483183024973186547867953777313232421875;-0.096537565963239924116123802377842366695404052734375;-0.057321807043975082918141339405337930656969547271728515625;-0.33528888680619395312731967351282946765422821044921875;0.254536930512510084501087703756638802587985992431640625;0.160443440271881343495152805189718492329120635986328125;0.0298865770847444554847438524802782922051846981048583984375;-0.4905367415926971119688460021279752254486083984375;0.26949914824714371608394003487774170935153961181640625;0.279888712410184592460637986732763238251209259033203125;0.156475783700833093181614685818203724920749664306640625;0.427246473409241656060686409546178765594959259033203125;0.24892939455984686158984686699113808572292327880859375;0.2130922585627052778800560872696223668754100799560546875;0.09388320364746434443237177447372232563793659210205078125;-0.159198518445238190732737848520628176629543304443359375;0.01438968371043083081806113199263563728891313076019287109375;-0.0623226293562786637370010112135787494480609893798828125;0.403201394446350114275645637462730519473552703857421875;-1.209114934242264904895591826061718165874481201171875;0.8556447732028324981712330554728396236896514892578125;-0.124638437957925785060098178291809745132923126220703125;-0.87136147182802703436976798911928199231624603271484375;0.68733337340105526980238437317893840372562408447265625;0.08171188805447136827009302351143560372292995452880859375;0.62154317245998480512270134568098001182079315185546875;-0.142201082792390798292814224623725749552249908447265625;-0.058134677163346359929363416085834614932537078857421875;-0.0164424917618185388590301698741313884966075420379638671875;0.0377358747014499840144452491585980169475078582763671875;0.292289912994841805105039611589745618402957916259765625;0.76420559375889940412207579356618225574493408203125;-0.03434516763233952385547809171839617192745208740234375;-0.037602080927664947862520961052723578177392482757568359375;0.006550485557210122648796879474275556276552379131317138671875;0.04940602468184761286718043038490577600896358489990234375;-0.1541501906398750343374359772496973164379596710205078125;0.01187461167243125149950433439016705960966646671295166015625;0.01447827447317109363089659979095813469029963016510009765625;0.0172233274061301920576649848726447089575231075286865234375]
      mask Display: e = 0.06;c1 = [120 150 230]/255;c2 = ([120 150 230]+0)/383;c3 = ([120 150 230]+128)/383;patch([0 1 1 0],[0 0 1 1],c1);patch([0 1 1 1-e 1-e 0+e],[0 0 1 1-e 0+e 0+e],c2);patch([0 0 1 1-e 0+e 0+e],[0 1 1 1-e 1-e 0+e],c3);plot([0 1 1 0 0],[0 0 1 1 0]);disp('weights');
  Mux : Mux  Inputs=1
      mask Display: e = 0.06;c1 = [120 150 230]/255;c2 = ([120 150 230]+0)/383;c3 = ([120 150 230]+128)/383;patch([0 1 1 0],[0 0 1 1],c1);patch([0 1 1 1-e 1-e 0+e],[0 0 1 1-e 0+e 0+e],c2);patch([0 0 1 1-e 0+e 0+e],[0 1 1 1-e 1-e 0+e],c3);plot([0 1 1 0 0],[0 0 1 1 0]);disp('Mux');
  dotprod1 : neural/Weight Functions/dotprod
  "lz{2,1}" : Outport
      mask Display: e = 0.06;c1 = [120 230 180]/255;c2 = ([120 230 180]+0)/(256+128);c3 = ([120 230 180]+128)/(256+128);patch([0 1 1 0],[0 0 1 1],c1);patch([0 1 1 1-e 1-e 0+e],[0 0 1 1-e 0+e 0+e],c2);patch([0 0 1 1-e 0+e 0+e],[0 1 1 1-e 1-e 0+e],c3);plot([0 1 1 0 0],[0 0 1 1 0]);
  wires:
  "IW{2,1}(1,:)'"/1 -> dotprod1/1
  "ad{2,1}"/1 -> dotprod1/2
  dotprod1/1 -> Mux/1
  Mux/1 -> "lz{2,1}"/1

== system mrefrobotarm_modified_previous_y_previous_u_previous_ref_pert/m=0.01 sd =0.01/Layer 1/Delays 1 ==
  "p{1}" : Inport  PortDimensions=10
      mask Display: e = 0.06;c1 = [120 230 180]/255;c2 = ([120 230 180]+0)/(256+128);c3 = ([120 230 180]+128)/(256+128);patch([0 1 1 0],[0 0 1 1],c1);patch([0 1 1 1-e 1-e 0+e],[0 0 1 1-e 0+e 0+e],c2);patch([0 0 1 1-e 0+e 0+e],[0 1 1 1-e 1-e 0+e],c3);plot([0 1 1 0 0],[0 0 1 1 0]);
  mux : Mux  Inputs=1
      mask Display: e = 0.06;c1 = [120 150 230]/255;c2 = ([120 150 230]+0)/383;c3 = ([120 150 230]+128)/383;patch([0 1 1 0],[0 0 1 1],c1);patch([0 1 1 1-e 1-e 0+e],[0 0 1 1-e 0+e 0+e],c2);patch([0 0 1 1-e 0+e 0+e],[0 1 1 1-e 1-e 0+e],c3);plot([0 1 1 0 0],[0 0 1 1 0]);disp('Mux')
  "pd{1,1}" : Outport
      mask Display: e = 0.06;c1 = [120 230 180]/255;c2 = ([120 230 180]+0)/(256+128);c3 = ([120 230 180]+128)/(256+128);patch([0 1 1 0],[0 0 1 1],c1);patch([0 1 1 1-e 1-e 0+e],[0 0 1 1-e 0+e 0+e],c2);patch([0 0 1 1-e 0+e 0+e],[0 1 1 1-e 1-e 0+e],c3);plot([0 1 1 0 0],[0 0 1 1 0]);
  wires:
  "p{1}"/1 -> mux/1
  mux/1 -> "pd{1,1}"/1
